simulink model "Standing_IE_Plat"  (R2019a)
settings: Solver=FixedStepAuto  StartTime=0.0  StopTime=400  FixedStep=Ts  RelTol=1e-3  EnableMultiTasking=on
InitFcn:
  | WEIGHT_TRIGGER_THRESHOLD = 20;
  | MAX_DISPLAY_WEIGHT = 40;
  | CENTER_VOLTAGE_WEIGHT = 2.5;
  | CENTER_VOLTAGE_DP_COP = 2.5;
  | CENTER_VOLTAGE_IE_COP = 2.5;
  | WEIGHT_VOLTAGE_OFFSET = 0.08;
  | DP_COP_VOLTAGE_OFFSET = 0.127;
  | IE_COP_VOLTAGE_OFFSET = 0.127;
  | VOLTAGE_BOUND = 2.0;
  | MAX_DISPLAY_COP_DP = 0.109;
  | MAX_DISPLAY_COP_IE = 0.109;
values from neighbouring files (symbols this model uses):
  DPbase = 0    [msstudy.m]    (also in mvc_reflex.m = nanmean(tsmovavg(Input3.data(1:20000,7),'s',1000,1)))
  DPF = (DP_cop)*(tweight)*0.01    [msstudy.m]
  f1_off = 0    [msstudy.m]    (also in pbase_l.m = nanmean(tsmovavg(Input3.data(1:40000,1),'s',1000,1)))
  f2_off = 0    [msstudy.m]    (also in pbase_l.m = nanmean(tsmovavg(Input3.data(1:40000,2),'s',1000,1)))
  f3_off = 0    [msstudy.m]    (also in pbase_l.m = nanmean(tsmovavg(Input3.data(1:40000,3),'s',1000,1)))
  f4_off = 0    [msstudy.m]    (also in pbase_l.m = nanmean(tsmovavg(Input3.data(1:40000,4),'s',1000,1)))
  f5_off = 0    [msstudy.m]    (also in pbase_l.m = nanmean(tsmovavg(Input3.data(1:40000,5),'s',1000,1)))
  f6_off = 0    [msstudy.m]    (also in pbase_l.m = nanmean(tsmovavg(Input3.data(1:40000,6),'s',1000,1)))
  forrange = 5    [msstudy.m]
  IEF = (CoP+IE_cop)*tweight*0.01    [msstudy.m]
  off_TA = 0    [msstudy.m]    (also in mvc_reflex.m = nanmean(tsmovavg(Input3.data(1:20000,1),'s',1000,1)))
  TA_MVC = 1    [msstudy.m]    (also in mvc_reflex.m = max((tsmovavg(abs(Input3.data(:,1)-off_TA),'s',1000,1))))
  trial = 1    [msstudy.m]
  Ts = 0.0005    [msstudy.m]
  tweight = 50*0.01*weight    [msstudy.m]    (also in weightcalc.m = weight/2)
undefined symbols (not defined in the file or in its folder): Pull, single_weight, up
libraries: speedgoatlib_IO183 x7, dspsigops x4, powerlib_meascontrol x3, slrtlib x3, dspswit3 x1, simulink x1
settings Model: Creator=vnalam  LastModifiedBy=vnalam
settings DataIOCC: LimitDataPoints=on  SaveFormat=StructureWithTime  ReturnWorkspaceOutputs=off
settings OptimizationCC: BlockReduction=off  OptimizeBlockIOStorage=off  BufferReuse=off  GlobalBufferReuse=off  ExpressionFolding=off  LocalBlockOutputs=off  LifeSpan=inf  OptimizeDataStoreBuffers=off  BusAssignmentInplaceUpdate=off
settings DebuggingCC: AllowSymbolicDim=off  SFUnexpectedBacktrackingDiag=warning  SFNoUnconditionalDefaultTransitionDiag=warning  SFExecutionAtInitializationDiag=none  ArithmeticOperatorsInVariantConditions=warning
settings HardwareCC: ProdBitPerPointer=32  ProdBitPerSizeT=32  ProdBitPerPtrDiffT=32  ProdLargestAtomicFloat=None  ProdWordSize=32  ProdLongLongMode=on  ProdHWDeviceType=Generic->32-bit x86 compatible
settings ModelReferenceCC: PropagateSignalLabelsOutOfModel=off
settings SFSimCC: SimUseLocalCustomCode=off
settings RTWCC: SystemTargetFile=slrt.tlc  TLCOptions=-axPCModelStackSizeKB=512  TemplateMakefile=slrt_default_tmf  Description=Simulink Real-Time  RTWUseLocalCustomCode=off  CodeExecutionProfiling=on  RTWCompilerOptimization=on
settings CodeAppCC: StateflowObjectComments=on
settings SimulinkRealTimeCC: PreserveStateflowLocalDataDimensions=off  RL32LogTETModifier=off  xPCConcurrentTasks=on
settings ConfigComp: CovMetricSettings=dw  CovHtmlReporting=on  CovSaveCumulativeToWorkspaceVar=on  CovSaveSingleToWorkspaceVar=on  CovExternalEMLEnable=off

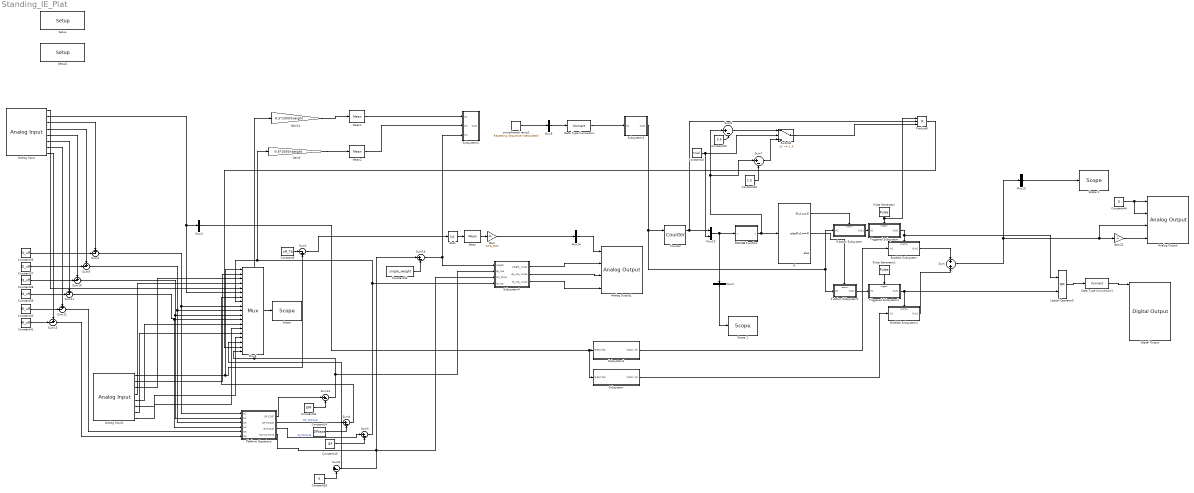
== system Standing_IE_Plat ==
  Abs1 : Abs
  Analog Input : speedgoatlib_IO183/Analog Input  Priority=0  parModuleId=1  parSampTime=Ts  parPciSlot=-1  parAdChannelLow=1  parAdChannelHigh=8
      settings: SourceProductName=Simulink Real-Time: Speedgoat Library
  Analog Input1 : speedgoatlib_IO183/Analog Input  Priority=0  parModuleId=2  parSampTime=Ts  parPciSlot=-1  parAdChannelLow=1  parAdChannelHigh=8
      settings: SourceProductName=Simulink Real-Time: Speedgoat Library
  Analog Output : speedgoatlib_IO183/Analog Output  parModuleId=1  parSampTime=Ts  parDaSimult=on  parPciSlot=-1  parDaChannels=[1 2 3 4]  parDaInit=[0 0 0 0]  parDaReset=[0 0 0 0]
      settings: SourceProductName=Simulink Real-Time: Speedgoat Library
  Analog Output1 : speedgoatlib_IO183/Analog Output  parModuleId=2  parSampTime=-1  parDaSimult=on  parPciSlot=-1  parDaChannels=[1 2 3 4]  parDaInit=[0 0 0 0]  parDaReset=[0 0 0 0]
      settings: SourceProductName=Simulink Real-Time: Speedgoat Library
  Constant10 : Constant  Value=trial  SampleTime=Ts
  Constant14 : Constant  Value=DPbase  SampleTime=Ts
  Constant15 : Constant  Value=IEF  SampleTime=Ts
  Constant23 : Constant  Value=3.5  SampleTime=Ts
  Constant24 : Constant  Value=1.5  SampleTime=Ts
  Constant28 : Constant  Value=0  SampleTime=Ts
  Constant36 : Constant  Value=f1_off  SampleTime=Ts
  Constant37 : Constant  Value=f2_off  SampleTime=Ts
  Constant38 : Constant  Value=f3_off  SampleTime=Ts
  Constant39 : Constant  Value=f4_off  SampleTime=Ts
  Constant40 : Constant  Value=f5_off  SampleTime=Ts
  Constant41 : Constant  Value=f6_off  SampleTime=Ts
  Constant42 : Constant  Value=DPF  SampleTime=Ts
  Constant43 : Constant  Value=single_weight  SampleTime=Ts
  Constant44 : Constant  Value=0  SampleTime=Ts
  Constant5 : Constant  Value=off_TA  SampleTime=Ts
  Counter : dspswit3/Counter  Direction=Up  CountEvent=Rising edge  CounterSize=User defined  MaxCount=255  InitialCount=0  Output=Count and Hit  HitValue=32  ResetInput=on  SamplesPerFrame=1  Ts=1  CntDtype=double  HitDtype=Boolean
  Data Type Conversion : DataTypeConversion
  Data Type Conversion1 : DataTypeConversion
  Digital Output : speedgoatlib_IO183/Digital Output  parModuleId=2  parSampTime=Ts  parPciSlot=-1  parDoChannels=[1 2 3 4 5 6 7 8]  parDoInit=[0 0 0 0 0 0 0 0]  parDoReset=[1 1 1 1 1 1 1 1]
      settings: SourceProductName=Simulink Real-Time: Speedgoat Library
  Enabled Subsystem : Subsystem  TreatAsAtomicUnit=on
  Enabled Subsystem1 : Subsystem  TreatAsAtomicUnit=on
  Gain : Gain  Gain=1/TA_MVC
  Gain14 : Gain  Gain=-0.5*1000/tweight
  Gain22 : Gain  Gain=-1
  Gain6 : Gain  Gain=-0.5*1000/tweight
  If : If  IfExpression=u1==3  ElseIfExpressions=u1==4
  If Action Subsystem : Subsystem  TreatAsAtomicUnit=on
  If Action Subsystem1 : Subsystem  TreatAsAtomicUnit=on
  Logical Operator5 : Logic  Operator=OR  AllPortsSameDT=off  OutDataTypeStr=boolean
  MATLAB Function : MATLAB Function  TreatAsAtomicUnit=on
  Mean : powerlib_meascontrol/Measurements/Mean  Freq=2  Vinit=0  Ts=0
      settings: SourceProductName=Simscape Electrical
  Mean1 : powerlib_meascontrol/Measurements/Mean  Freq=2  Vinit=0  Ts=0
      settings: SourceProductName=Simscape Electrical
  Mean2 : powerlib_meascontrol/Measurements/Mean  Freq=2  Vinit=0  Ts=0
      settings: SourceProductName=Simscape Electrical
  Mux10 : Mux  Inputs=2
  Mux{2..3,9,14..15} (5 alike) : Mux  Inputs=1
  Mux6 : Mux  Inputs=19
      settings: DisplayOption=signals
  Platform Equations : Subsystem
  Product8 : Product  Inputs=3
  Pulse Generator : DiscretePulseGenerator  Period=2081  SampleTime=Ts
  Pulse Generator1 : DiscretePulseGenerator  Period=2081  SampleTime=Ts
  "Scope " : slrtlib/Displays and Logging/Scope   scopeno=3  scopetype=File  autostart=on  viewmode=Graphical redraw  formatstr='%15.6f'  grid=on  ylimits=[0,0]  nosamples=800000  noprepostsamples=0  interleave=1  triggermode=FreeRun  triggersignal=1  trigsignalfromport=off  triggerlevel=0.0  triggerslope=Either  triggerscope=1  triggersample=0  filename=XIEP.dat  mode=Commit  writesize=512  autorestart=off  dynamicfilemode=off  maxwritefilesize=512*1024^2
  Scope 1 : slrtlib/Displays and Logging/Scope   scopeno=1  scopetype=Target  autostart=on  viewmode=Numerical  formatstr='%15.6f'  grid=on  ylimits=[0,0]  nosamples=200  noprepostsamples=0  interleave=1  triggermode=FreeRun  triggersignal=1  trigsignalfromport=off  triggerlevel=0.0  triggerslope=Either  triggerscope=1  triggersample=0  filename=tot303.dat  mode=Lazy  writesize=512  autorestart=off  dynamicfilemode=off  maxwritefilesize=512*1024^2
  Scope 2 : slrtlib/Displays and Logging/Scope   scopeno=2  scopetype=Target  autostart=on  viewmode=Graphical rolling  formatstr='%15.6f'  grid=on  ylimits=[0,0]  nosamples=8000  noprepostsamples=0  interleave=1  triggermode=FreeRun  triggersignal=1  trigsignalfromport=off  triggerlevel=0.0  triggerslope=Either  triggerscope=1  triggersample=0  filename=tot303.dat  mode=Lazy  writesize=512  autorestart=off  dynamicfilemode=off  maxwritefilesize=512*1024^2
  Setup : speedgoatlib_IO183/Setup  parModuleId=1  parPciSlot=-1  parDaSimult=on  parAdCoupling=Single Ended  parAdRange=+-10V  parAdChannelLow=1  parAdChannelHigh=8  parDaChannels=[1:4]  parDaRange=0..5V  parDaInit=[0]  parDaReset=[0]  parDoChannels=[1:8]  parDoInit=[0]  parDoReset=[1]  parDiChannels=[9:16]  parIOPullReferenceFront=Pull-up (3.3V)  parIOPullReferenceRear=Pull-up (3.3V)
      settings: SourceProductName=Simulink Real-Time: Speedgoat Library
  Setup1 : speedgoatlib_IO183/Setup  parModuleId=2  parPciSlot=-1  parDaSimult=on  parAdCoupling=Single Ended  parAdRange=+-10V  parAdChannelLow=1  parAdChannelHigh=8  parDaChannels=[1:4]  parDaRange=0..5V  parDaInit=[0]  parDaReset=[0]  parDoChannels=[1:8]  parDoInit=[0]  parDoReset=[1]  parDiChannels=[9:16]  parIOPullReferenceFront=Pull-up (3.3V)  parIOPullReferenceRear=Pull-up (3.3V)
      settings: SourceProductName=Simulink Real-Time: Speedgoat Library
  Subsystem : Subsystem
  Subsystem1 : Subsystem
  Subsystem2 : Subsystem
  Subsystem3 : Subsystem
  Subsystem4 : Subsystem
  Sum : Sum  Inputs=+|+
  Sum1 : Sum  Inputs=|-+
  Sum{3,9..13} (6 alike) : Sum  Inputs=+-|
  Sum{4..8,14,16} (7 alike) : Sum  Inputs=|+-
  Switch8 : Switch  Threshold=1.5
  Triggered Subsystem : Subsystem  TreatAsAtomicUnit=on
  Triggered Subsystem1 : Subsystem  TreatAsAtomicUnit=on
  smoothened ramp2 : simulink/Sources/Repeating Sequence Interpolated  OutValues="[0 1 1 0  0 ].'"  TimeValues=[0 0.0001 1.001 1.002 4].'  LookUpMeth=Interpolation-Use End Values  tsamp=Ts  OutMin=[]  OutMax=[]  OutDataTypeStr=double  OutputDataTypeScalingMode=double  OutDataType=fixdt(0,8)  OutScaling=2^-10
  wires:
  Constant5/1 -> Sum1/1
  Mean/1 -> Gain/1
  Sum1/1 -> Abs1/1
  Abs1/1 -> Mean/1
  Pulse Generator/1 -> Product8/1, Triggered Subsystem/Trigger
  Triggered Subsystem/1(Out1) -> Enabled Subsystem/Enable, Logical Operator5/1
  Enabled Subsystem/1(Out1) -> Sum/1
  MATLAB Function/1(y) -> Sum6/1, Sum7/1, If/1
  Pulse Generator1/1 -> Triggered Subsystem1/Trigger
  Triggered Subsystem1/1(Out1) -> Enabled Subsystem1/Enable, Logical Operator5/2
  Enabled Subsystem1/1(Out1) -> Sum/2
  If Action Subsystem1/1(Out1) -> Triggered Subsystem1/1(In1)
  Mux9/1 -> Data Type Conversion/1
  If/1 -> If Action Subsystem/Action
  If/2 -> If Action Subsystem1/Action
  Counter/1 -> Product8/2, Mux10/1
  Constant14/1 -> Sum4/2
  Constant15/1 -> Sum5/2
  Sum5/1 -> Subsystem4/4(ie_cop), Gain6/1, Mux6/8
  Mean1/1 -> Subsystem2/1(In1)
  Subsystem4/2(dp_cop_visual) -> Analog Output1/3
  Mean2/1 -> Subsystem2/2(In2)
  Sum/1 -> Mux15/1, Analog Output/3, Gain22/1
  Gain14/1 -> Mean1/1
  Gain6/1 -> Mean2/1
  If Action Subsystem/1(Out1) -> Triggered Subsystem/1(In1)
  Logical Operator5/1 -> Data Type Conversion1/1
  Constant10/1 -> Mux10/2, Switch8/2
  Sum6/1 -> Switch8/1
  Sum7/1 -> Switch8/3
  Constant23/1 -> Sum6/2
  Constant24/1 -> Sum7/2
  Switch8/1 -> Product8/3
  Mux10/1 -> Mux2/1, MATLAB Function/1(u)
  Gain/1 -> Mux14/1
  Mux15/1 -> Scope 2/1
  Sum9/1 -> Mux6/10, Platform Equations/3(In3)
  Sum10/1 -> Mux6/11, Platform Equations/2(In2)
  Sum11/1 -> Mux6/12, Platform Equations/4(In4)
  Sum12/1 -> Platform Equations/5(In5)
  Sum13/1 -> Platform Equations/6(In6)
  Sum3/1 -> Mux6/9, Platform Equations/1(In1)
  Analog Input1/1 -> Sum1/2, Mux6/1
  Mux2/1 -> Scope 1/1
  Constant28/1 -> Sum8/2
  Mux3/1 -> Subsystem1/1(IE Enc Pos), Subsystem/1(IE Enc Pos)
  Analog Input/3 -> Sum3/1
  Analog Input/5 -> Sum10/1
  Analog Input/4 -> Sum9/1
  Analog Input/6 -> Sum11/1
  Constant36/1 -> Sum3/2
  Constant37/1 -> Sum9/2
  Constant38/1 -> Sum10/2
  Constant39/1 -> Sum11/2
  Analog Input/7 -> Sum12/1
  Constant40/1 -> Sum12/2
  Analog Input/8 -> Sum13/1
  Constant41/1 -> Sum13/2
  Constant42/1 -> Sum14/2
  Sum14/1 -> Subsystem4/2(dp_cop), Mux6/19, Gain14/1
  Constant43/1 -> Sum16/2
  Sum16/1 -> Subsystem4/1(weight), Subsystem2/3(In4)
  Mux14/1 -> Analog Output1/1
  Analog Input/1 -> Mux6/5
  Mux6/1 -> "Scope "/1
  Analog Input1/2 -> Mux6/2
  Analog Input1/3 -> Mux6/3
  Analog Input1/4 -> Mux6/4
  Analog Input/2 -> Mux3/1, Mux6/6
  Sum4/1 -> Mux6/7
  Analog Input1/5 -> Mux6/13
  Analog Input1/6 -> Mux6/14
  Analog Input1/7 -> Mux6/15
  Analog Input1/8 -> Mux6/16
  Product8/1 -> Mux6/18
  Sum8/1 -> Mux6/17
  Data Type Conversion1/1 -> Digital Output/1
  smoothened ramp2/1 -> Mux9/1
  Subsystem/1(Motor Vel) -> Enabled Subsystem1/1(In1)
  Subsystem1/1(Motor Vel) -> Enabled Subsystem/1(In1)
  Platform Equations/2(DP Torque) -> Sum4/1  "DP_TORQUE"
  Platform Equations/4(Normal Force) -> Subsystem4/3(act_force), Sum16/1, Sum8/1
  Platform Equations/3(IE Torque) -> Sum5/1  "IE_TORQUE"
  Platform Equations/1(DP COP?) -> Sum14/1
  Subsystem3/1(Out1) -> Counter/1, If Action Subsystem1/1(In1), If Action Subsystem/1(In1)
  Data Type Conversion/1 -> Subsystem3/1(In1)
  Gain22/1 -> Analog Output/4
  Constant44/1 -> Analog Output/2, Analog Output/1
  Subsystem4/3(ie_cop_visual) -> Analog Output1/4
  Subsystem4/1(weight_visual) -> Analog Output1/2

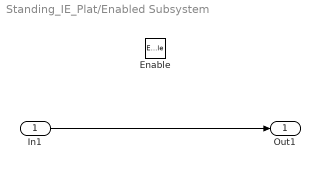
== system Standing_IE_Plat/Enabled Subsystem ==
  In1 : Inport
  Enable : EnablePort
  Out1 : Outport
  wires:
  In1/1 -> Out1/1

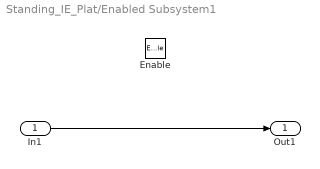
== system Standing_IE_Plat/Enabled Subsystem1 ==
  In1 : Inport
  Enable : EnablePort
  Out1 : Outport
  wires:
  In1/1 -> Out1/1

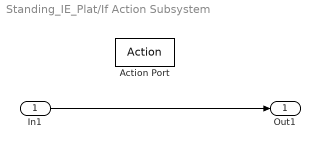
== system Standing_IE_Plat/If Action Subsystem ==
  In1 : Inport
  Action Port : ActionPort  ActionPortLabel=if(u1==3)
  Out1 : Outport
  wires:
  In1/1 -> Out1/1

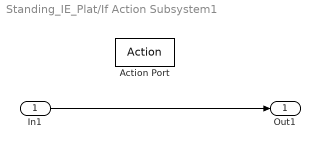
== system Standing_IE_Plat/If Action Subsystem1 ==
  In1 : Inport
  Action Port : ActionPort  ActionPortLabel=elseif(u1==4)
  Out1 : Outport
  wires:
  In1/1 -> Out1/1

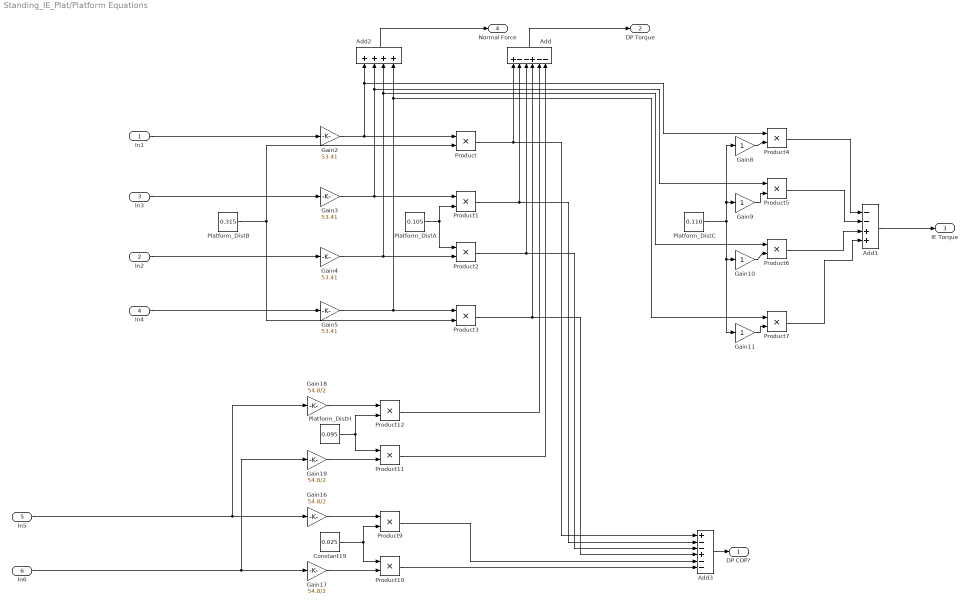
== system Standing_IE_Plat/Platform Equations ==
  In1 : Inport
  In2 : Inport  Port=2
  In3 : Inport  Port=3
  In4 : Inport  Port=4
  In5 : Inport  Port=5
  In6 : Inport  Port=6
  Add : Sum  Inputs=+--+--
  Add1 : Sum  Inputs=--++
  Add2 : Sum  Inputs=++++
  Add3 : Sum  Inputs=+--+--
  Constant19 : Constant  Value=0.025  SampleTime=-1
  Gain{8..11} (4 alike) : Gain
  Gain{16..19} (4 alike) : Gain  Gain=54.8/2
  Gain{2..5} (4 alike) : Gain  Gain=53.41
  Platform_DistA : Constant  Value=0.105  SampleTime=-1
  Platform_DistB : Constant  Value=0.315  SampleTime=-1
  Platform_DistC : Constant  Value=0.110  SampleTime=-1
  Platform_DistH : Constant  Value=0.095  SampleTime=-1
  Product{,1..7,9..12} (12 alike) : Product
  DP COP? : Outport
  DP Torque : Outport  Port=2
  IE Torque : Outport  Port=3
  Normal Force : Outport  Port=4
  wires:
  Product6/1 -> Add1/3
  Gain3/1 -> Product5/1, Add2/2, Product1/1
  Product9/1 -> Add3/5
  Product10/1 -> Add3/6
  Product/1 -> Add/1, Add3/1
  Add1/1 -> IE Torque/1
  Add2/1 -> Normal Force/1
  Platform_DistA/1 -> Product2/1, Product1/2
  Platform_DistH/1 -> Product11/1, Product12/2
  Gain9/1 -> Product5/2
  Gain5/1 -> Product3/1, Product7/1, Add2/4
  In5/1 -> Gain16/1, Gain18/1
  Platform_DistC/1 -> Gain8/1, Gain9/1, Gain11/1, Gain10/1
  Gain2/1 -> Product/1, Product4/1, Add2/1
  Gain18/1 -> Product12/1
  Gain10/1 -> Product6/2
  Product2/1 -> Add3/3, Add/3
  Add/1 -> DP Torque/1
  Platform_DistB/1 -> Product3/2, Product/2
  In6/1 -> Gain17/1, Gain19/1
  In3/1 -> Gain3/1
  Product4/1 -> Add1/1
  Product3/1 -> Add3/4, Add/4
  Gain11/1 -> Product7/2
  Gain4/1 -> Product2/2, Product6/1, Add2/3
  Product11/1 -> Add/6
  Product12/1 -> Add/5
  Product5/1 -> Add1/2
  In1/1 -> Gain2/1
  Product1/1 -> Add/2, Add3/2
  Add3/1 -> DP COP?/1
  Gain8/1 -> Product4/2
  Gain16/1 -> Product9/1
  Product7/1 -> Add1/4
  In2/1 -> Gain4/1
  In4/1 -> Gain5/1
  Gain17/1 -> Product10/2
  Constant19/1 -> Product9/2, Product10/1
  Gain19/1 -> Product11/2

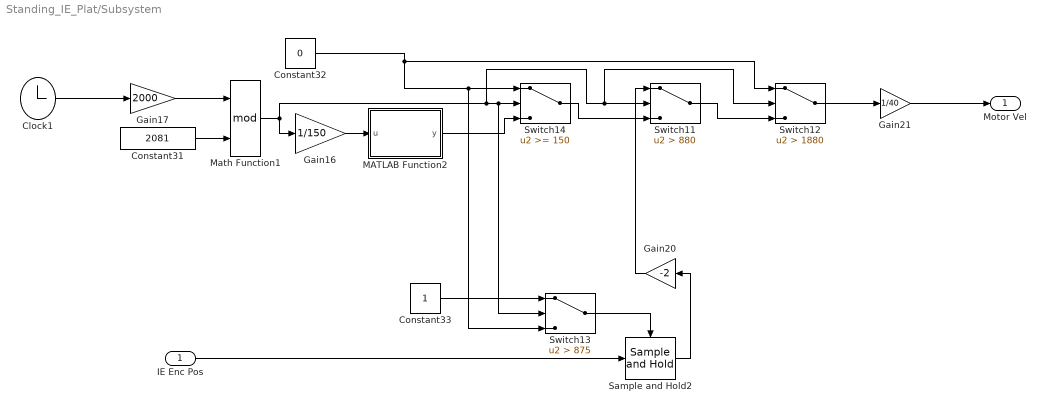
== system Standing_IE_Plat/Subsystem ==
  IE Enc Pos : Inport
  Clock1 : Clock
  Constant31 : Constant  Value=2081
  Constant32 : Constant  Value=0  SampleTime=Ts
  Constant33 : Constant  SampleTime=Ts
  Gain16 : Gain  Gain=1/150
  Gain17 : Gain  Gain=2000
  Gain20 : Gain  Gain=-2
  Gain21 : Gain  Gain=1/40
  MATLAB Function2 : MATLAB Function  TreatAsAtomicUnit=on
  Math Function1 : Math  Operator=mod  OutputSignalType=real  SaturateOnIntegerOverflow=on
  Sample and Hold2 : dspsigops/Sample and Hold  trig=Rising edge  initCond=0  latchinput=off
  Switch11 : Switch  Criteria=u2 > Threshold  Threshold=880
  Switch12 : Switch  Criteria=u2 > Threshold  Threshold=1880
  Switch13 : Switch  Criteria=u2 > Threshold  Threshold=875
  Switch14 : Switch  Threshold=150
  Motor Vel : Outport  VectorParamsAs1DForOutWhenUnconnected=on
  wires:
  Switch11/1 -> Switch12/3
  Constant31/1 -> Math Function1/2
  Gain20/1 -> Switch11/1
  Clock1/1 -> Gain17/1
  Switch14/1 -> Switch11/3
  MATLAB Function2/1(y) -> Switch14/3
  IE Enc Pos/1 -> Sample and Hold2/1
  Gain16/1 -> MATLAB Function2/1(u)
  Constant33/1 -> Switch13/1
  Math Function1/1 -> Gain16/1, Switch12/2, Switch11/2, Switch13/2, Switch14/2
  Gain17/1 -> Math Function1/1
  Sample and Hold2/1 -> Gain20/1
  Gain21/1 -> Motor Vel/1
  Switch13/1 -> Sample and Hold2/Trigger
  Constant32/1 -> Switch12/1, Switch13/3, Switch14/1
  Switch12/1 -> Gain21/1

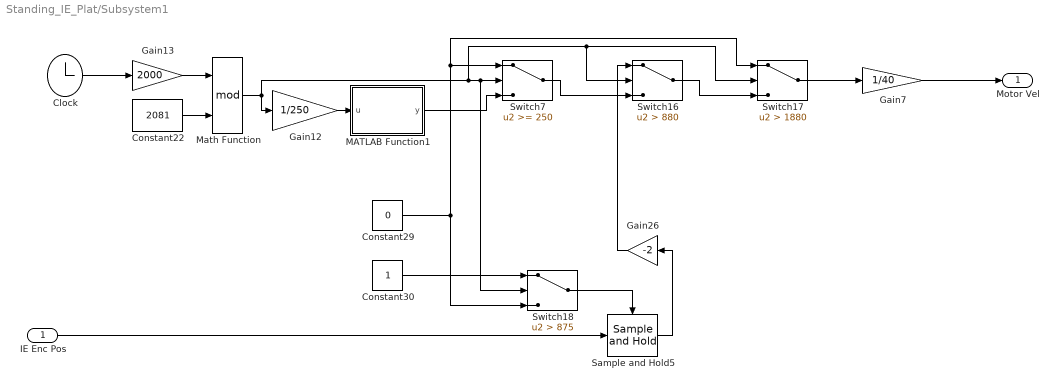
== system Standing_IE_Plat/Subsystem1 ==
  IE Enc Pos : Inport
  Clock : Clock
  Constant22 : Constant  Value=2081
  Constant29 : Constant  Value=0  SampleTime=Ts
  Constant30 : Constant  SampleTime=Ts
  Gain12 : Gain  Gain=1/250
  Gain13 : Gain  Gain=2000
  Gain26 : Gain  Gain=-2
  Gain7 : Gain  Gain=1/40
  MATLAB Function1 : MATLAB Function  TreatAsAtomicUnit=on
  Math Function : Math  Operator=mod  OutputSignalType=real  SaturateOnIntegerOverflow=on
  Sample and Hold5 : dspsigops/Sample and Hold  trig=Rising edge  initCond=0  latchinput=off
  Switch16 : Switch  Criteria=u2 > Threshold  Threshold=880
  Switch17 : Switch  Criteria=u2 > Threshold  Threshold=1880
  Switch18 : Switch  Criteria=u2 > Threshold  Threshold=875
  Switch7 : Switch  Threshold=250
  Motor Vel : Outport  VectorParamsAs1DForOutWhenUnconnected=on
  wires:
  Gain12/1 -> MATLAB Function1/1(u)
  Gain13/1 -> Math Function/1
  Constant30/1 -> Switch18/1
  IE Enc Pos/1 -> Sample and Hold5/1
  Constant22/1 -> Math Function/2
  MATLAB Function1/1(y) -> Switch7/3
  Math Function/1 -> Gain12/1, Switch16/2, Switch17/2, Switch18/2, Switch7/2
  Gain26/1 -> Switch16/1
  Clock/1 -> Gain13/1
  Gain7/1 -> Motor Vel/1
  Switch17/1 -> Gain7/1
  Switch16/1 -> Switch17/3
  Constant29/1 -> Switch7/1, Switch17/1, Switch18/3
  Switch18/1 -> Sample and Hold5/Trigger
  Sample and Hold5/1 -> Gain26/1
  Switch7/1 -> Switch16/3

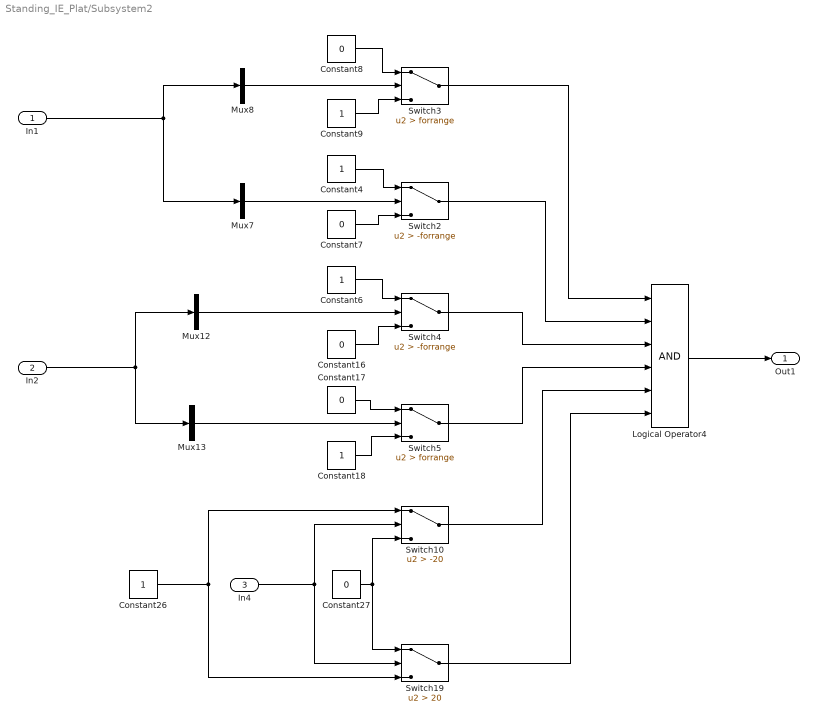
== system Standing_IE_Plat/Subsystem2 ==
  In1 : Inport
  In2 : Inport  Port=2
  In4 : Inport  Port=3
  Constant{7..8,16..17,27} (5 alike) : Constant  Value=0  SampleTime=Ts
  Constant{4,6,9,18,26} (5 alike) : Constant  SampleTime=Ts
  Logical Operator4 : Logic  Inputs=6  AllPortsSameDT=off  OutDataTypeStr=boolean
  Mux{7..8,12..13} (4 alike) : Mux  Inputs=1
  Switch10 : Switch  Criteria=u2 > Threshold  Threshold=-20
  Switch19 : Switch  Criteria=u2 > Threshold  Threshold=20
  Switch2 : Switch  Criteria=u2 > Threshold  Threshold=-forrange
  Switch3 : Switch  Criteria=u2 > Threshold  Threshold=forrange
  Switch4 : Switch  Criteria=u2 > Threshold  Threshold=-forrange
  Switch5 : Switch  Criteria=u2 > Threshold  Threshold=forrange
  Out1 : Outport  VectorParamsAs1DForOutWhenUnconnected=on
  wires:
  Constant9/1 -> Switch3/3
  Constant17/1 -> Switch5/1
  Mux13/1 -> Switch5/2
  Switch2/1 -> Logical Operator4/2
  In1/1 -> Mux7/1, Mux8/1
  Mux7/1 -> Switch2/2
  In2/1 -> Mux13/1, Mux12/1
  Constant4/1 -> Switch2/1
  Logical Operator4/1 -> Out1/1
  Switch10/1 -> Logical Operator4/5
  In4/1 -> Switch10/2, Switch19/2
  Constant16/1 -> Switch4/3
  Constant18/1 -> Switch5/3
  Switch5/1 -> Logical Operator4/4
  Constant26/1 -> Switch19/3, Switch10/1
  Constant8/1 -> Switch3/1
  Switch3/1 -> Logical Operator4/1
  Constant7/1 -> Switch2/3
  Mux12/1 -> Switch4/2
  Mux8/1 -> Switch3/2
  Constant6/1 -> Switch4/1
  Switch19/1 -> Logical Operator4/6
  Switch4/1 -> Logical Operator4/3
  Constant27/1 -> Switch19/1, Switch10/3

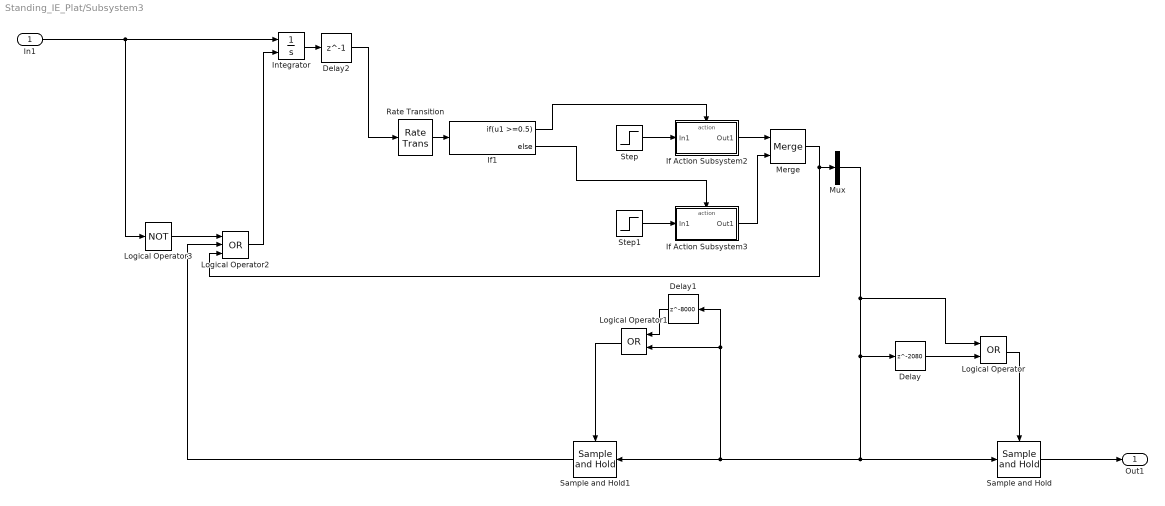
== system Standing_IE_Plat/Subsystem3 ==
  In1 : Inport
  Delay : Delay  DelayLength=2080  InitialCondition=0  SampleTime=Ts
  Delay1 : Delay  DelayLength=8000  InitialCondition=0  SampleTime=Ts
  Delay2 : Delay  DelayLength=1  InitialCondition=0  SampleTime=Ts
  If Action Subsystem2 : Subsystem  TreatAsAtomicUnit=on
  If Action Subsystem3 : Subsystem  TreatAsAtomicUnit=on
  If1 : If  IfExpression=u1 >=0.5
  Integrator : Integrator  ExternalReset=level hold
  Logical Operator : Logic  Operator=OR  AllPortsSameDT=off  OutDataTypeStr=boolean
  Logical Operator1 : Logic  Operator=OR  AllPortsSameDT=off  OutDataTypeStr=boolean
  Logical Operator2 : Logic  Operator=OR  Inputs=3  AllPortsSameDT=off  OutDataTypeStr=boolean
  Logical Operator3 : Logic  Operator=NOT  AllPortsSameDT=off  OutDataTypeStr=boolean
  Merge : Merge  InitialOutput=0
  Mux : Mux  Inputs=1
  Rate Transition : RateTransition  OutPortSampleTime=Ts
  Sample and Hold : dspsigops/Sample and Hold  trig=Rising edge  initCond=0  latchinput=off
  Sample and Hold1 : dspsigops/Sample and Hold  trig=Rising edge  initCond=0  latchinput=off
  Step : Step  Before=1  SampleTime=Ts
  Step1 : Step  After=0  SampleTime=Ts
  Out1 : Outport  VectorParamsAs1DForOutWhenUnconnected=on
  wires:
  If1/2 -> If Action Subsystem3/Action
  Logical Operator2/1 -> Integrator/2
  Sample and Hold1/1 -> Logical Operator2/2
  If Action Subsystem2/1(Out1) -> Merge/1
  Logical Operator/1 -> Sample and Hold/Trigger
  Sample and Hold/1 -> Out1/1
  Merge/1 -> Logical Operator2/3, Mux/1
  In1/1 -> Integrator/1, Logical Operator3/1
  Step1/1 -> If Action Subsystem3/1(In1)
  Mux/1 -> Delay1/1, Logical Operator1/2, Sample and Hold1/1, Sample and Hold/1, Delay/1, Logical Operator/1
  If1/1 -> If Action Subsystem2/Action
  Logical Operator1/1 -> Sample and Hold1/Trigger
  Integrator/1 -> Delay2/1
  Rate Transition/1 -> If1/1
  Delay2/1 -> Rate Transition/1
  Delay/1 -> Logical Operator/2
  Delay1/1 -> Logical Operator1/1
  Step/1 -> If Action Subsystem2/1(In1)
  If Action Subsystem3/1(Out1) -> Merge/2
  Logical Operator3/1 -> Logical Operator2/1

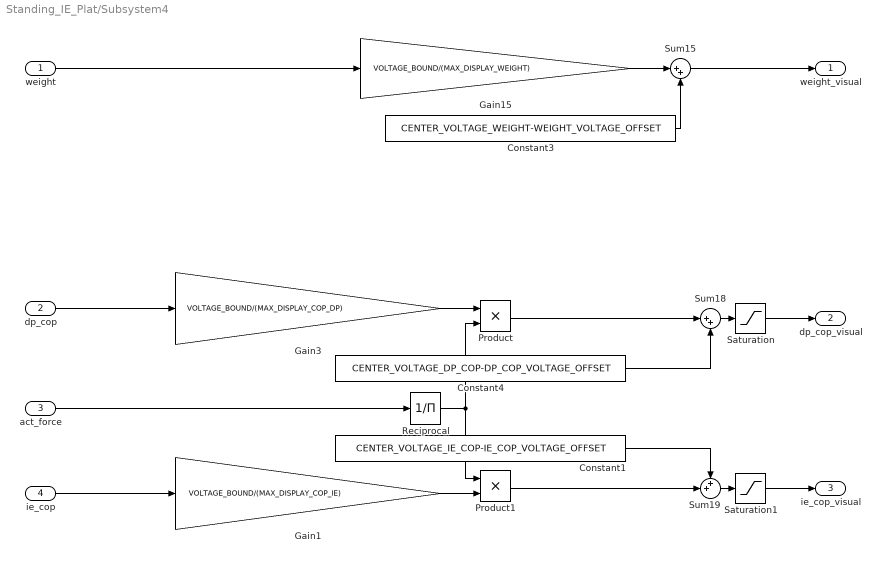
== system Standing_IE_Plat/Subsystem4 ==
  weight : Inport
  dp_cop : Inport  Port=2
  act_force : Inport  Port=3
  ie_cop : Inport  Port=4
  Constant1 : Constant  Value=CENTER_VOLTAGE_IE_COP-IE_COP_VOLTAGE_OFFSET  SampleTime=Ts
  Constant3 : Constant  Value=CENTER_VOLTAGE_WEIGHT-WEIGHT_VOLTAGE_OFFSET  SampleTime=Ts
  Constant4 : Constant  Value=CENTER_VOLTAGE_DP_COP-DP_COP_VOLTAGE_OFFSET  SampleTime=Ts
  Gain1 : Gain  Gain=VOLTAGE_BOUND/(MAX_DISPLAY_COP_IE)
  Gain15 : Gain  Gain=VOLTAGE_BOUND/(MAX_DISPLAY_WEIGHT)
  Gain3 : Gain  Gain=VOLTAGE_BOUND/(MAX_DISPLAY_COP_DP)
  Product : Product
  Product1 : Product
  Reciprocal : Product  Inputs=/
  Saturation : Saturate  UpperLimit=5.0  LowerLimit=0
  Saturation1 : Saturate  UpperLimit=5.0  LowerLimit=0
  Sum15 : Sum  Inputs=|++
  Sum18 : Sum  Inputs=|++
  Sum19 : Sum  Inputs=++|
  weight_visual : Outport
  dp_cop_visual : Outport  Port=2
  ie_cop_visual : Outport  Port=3
  wires:
  Constant1/1 -> Sum19/1
  Constant3/1 -> Sum15/2
  Reciprocal/1 -> Product/2, Product1/1
  Gain1/1 -> Product1/2
  Product1/1 -> Sum19/2
  Gain15/1 -> Sum15/1
  Product/1 -> Sum18/1
  Sum19/1 -> Saturation1/1
  act_force/1 -> Reciprocal/1
  Constant4/1 -> Sum18/2
  Sum18/1 -> Saturation/1
  Gain3/1 -> Product/1
  Sum15/1 -> weight_visual/1
  Saturation1/1 -> ie_cop_visual/1
  ie_cop/1 -> Gain1/1
  Saturation/1 -> dp_cop_visual/1
  dp_cop/1 -> Gain3/1
  weight/1 -> Gain15/1

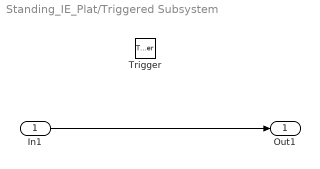
== system Standing_IE_Plat/Triggered Subsystem ==
  In1 : Inport
  Trigger : TriggerPort  VariantControl=(inherit)
  Out1 : Outport
  wires:
  In1/1 -> Out1/1

== system Standing_IE_Plat/Triggered Subsystem1 ==
  In1 : Inport
  Trigger : TriggerPort  VariantControl=(inherit)
  Out1 : Outport
  wires:
  In1/1 -> Out1/1

== system Standing_IE_Plat/Subsystem3/If Action Subsystem2 ==
  In1 : Inport
  Action Port : ActionPort  ActionPortLabel=if(u1 >=0.5)
  Out1 : Outport
  wires:
  In1/1 -> Out1/1

== system Standing_IE_Plat/Subsystem3/If Action Subsystem3 ==
  In1 : Inport
  Action Port : ActionPort  ActionPortLabel=else
  Out1 : Outport
  wires:
  In1/1 -> Out1/1

== matlab function Standing_IE_Plat/Subsystem1/MATLAB Function1 ==
  data: u input; y output
function y = fcn(u)
%#codegen
y=3*((30*u^2-60*u^3+30*u^4))*2000/250;

== matlab function Standing_IE_Plat/MATLAB Function ==
  data: u input; y output
function y = fcn(u)
%#codegen
y=0;

    
    if u(1)==1
        y=3;
    elseif u(1)==2
        y=3;
    elseif u(1)==3
        y=3;
    elseif u(1)==4
        y=3;
    elseif u(1)==5
        y=3;
    elseif u(1)==6
        y=3;
    elseif u(1)==7
        y=3;
    elseif u(1)==8
        y=3;
    elseif u(1)==9
        y=3;
    elseif u(1)==10
        y=3;

  
    else
        y=0;
    end
end

== matlab function Standing_IE_Plat/Subsystem/MATLAB Function2 ==
  data: u input; y output
function y = fcn(u)
%#codegen
y=-3*((30*u^2-60*u^3+30*u^4))*2000/150;
